simulink model "exp5_2"  (R2019a)
settings: Solver=VariableStepAuto  StartTime=0.0  StopTime=20  RelTol=1e-3
settings Model: Creator=83621  LastModifiedBy=83621

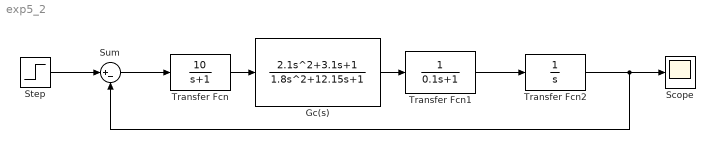
== system exp5_2 ==
  Gc(s) : TransferFcn  Numerator=[2.1 3.1 1]  Denominator=[1.8 12.15 1]
  Scope : Scope
  Step : Step  SampleTime=0
  Sum : Sum  Inputs=|+-
  Transfer Fcn : TransferFcn  Numerator=[10]  Denominator=[1 1]
  Transfer Fcn1 : TransferFcn  Denominator=[0.1 1]
  Transfer Fcn2 : TransferFcn  Denominator=[1 0]
  wires:
  Sum/1 -> Transfer Fcn/1
  Step/1 -> Sum/1
  Transfer Fcn2/1 -> Sum/2, Scope/1
  Gc(s)/1 -> Transfer Fcn1/1
  Transfer Fcn/1 -> Gc(s)/1
  Transfer Fcn1/1 -> Transfer Fcn2/1
